simulink model "Sim5_MMC"  (R2019a)
settings: Solver=ode1  StartTime=0.0  StopTime=4  FixedStep=Time_Step  RelTol=1e-3
undefined symbols (not defined in the file): DiscIntNeverNeededParam, GRD00_Lg, GRD00_Rg, Time_Step, VSC01_id0
libraries: powerlib x107, Control_Lib x16, simulink x15, spsCurrentMeasurementLib x14, powerlib_meascontrol x4
(part 3 of 5)

== system Sim5_MMC/CCSC/Control loops/Power Control Loops ==
  P_mes : Inport
  P_set : Inport  Port=2
  delta_PLL : Inport  Port=3
  w_PLL : Inport  Port=4
  Compare To Constant : simulink/Logic and Bit Operations/Compare To Constant  relop===  const=1  OutDataTypeStr=boolean
  Compare To Constant1 : simulink/Logic and Bit Operations/Compare To Constant  relop===  const=2  OutDataTypeStr=boolean
  Compare To Constant2 : simulink/Logic and Bit Operations/Compare To Constant  relop===  const=3  OutDataTypeStr=boolean
  Inertia Less : Subsystem
  Multiport Switch : MultiPortSwitch
  Multiport Switch1 : MultiPortSwitch
  Mux : Mux  Inputs=[1 1]
  PI Controler : Subsystem
  Trigonometric Function : Trigonometry  Operator=cos
  Trigonometric Function1 : Trigonometry
  VSM : Subsystem
  w_set{1..4} (4 alike) : Constant  Value=Chosen_Strategy
  w_set_pu : Constant
  f : Outport  PortDimensions=1  VectorParamsAs1DForOutWhenUnconnected=off
  Theta : Outport  Port=2  VectorParamsAs1DForOutWhenUnconnected=off
  CosSinTheta : Outport  Port=3  PortDimensions=2  VectorParamsAs1DForOutWhenUnconnected=off
  wires:
  Multiport Switch1/1 -> Trigonometric Function1/1, Trigonometric Function/1, Theta/1
  Trigonometric Function1/1 -> Mux/2
  Mux/1 -> CosSinTheta/1
  Trigonometric Function/1 -> Mux/1
  Compare To Constant2/1 -> PI Controler/Enable
  Compare To Constant1/1 -> VSM/Enable
  Compare To Constant/1 -> Inertia Less/Enable
  w_set4/1 -> Compare To Constant2/1
  w_set2/1 -> Compare To Constant1/1
  w_set3/1 -> Compare To Constant/1
  Inertia Less/1(frequency) -> Multiport Switch/2
  Multiport Switch/1 -> f/1
  Inertia Less/2(theta) -> Multiport Switch1/2
  VSM/2(theta) -> Multiport Switch1/3
  w_set1/1 -> Multiport Switch/1, Multiport Switch1/1
  VSM/1(frequency) -> Multiport Switch/3
  PI Controler/1(frequency) -> Multiport Switch/4
  PI Controler/2(theta) -> Multiport Switch1/4
  w_set_pu/1 -> PI Controler/3(w_set_pu)
  w_PLL/1 -> Inertia Less/4(w_PLL), VSM/3(w_PLL)
  delta_PLL/1 -> Inertia Less/3(delta_PLL)
  P_set/1 -> Inertia Less/2(P_set), VSM/2(P_set), PI Controler/2(P_set)
  P_mes/1 -> Inertia Less/1(P_mes), VSM/1(P_mes), PI Controler/1(P_mes)

== system Sim5_MMC/CCSC/Control loops/Power Control Loops1 ==
  P_mes : Inport
  P_set : Inport  Port=2
  delta_PLL : Inport  Port=3
  w_PLL : Inport  Port=4
  Delta_E_dq : Inport  Port=5
  Compare To Constant : simulink/Logic and Bit Operations/Compare To Constant  relop===  const=1  OutDataTypeStr=boolean
  Compare To Constant1 : simulink/Logic and Bit Operations/Compare To Constant  relop===  const=2  OutDataTypeStr=boolean
  Compare To Constant2 : simulink/Logic and Bit Operations/Compare To Constant  relop===  const=3  OutDataTypeStr=boolean
  Inertia Less : Subsystem
  Multiport Switch : MultiPortSwitch
  Multiport Switch1 : MultiPortSwitch
  Mux : Mux  Inputs=[1 1]
  PI Controler : Subsystem
  Subsystem : Subsystem
  Trigonometric Function : Trigonometry  Operator=cos
  Trigonometric Function1 : Trigonometry
  VSM : Subsystem
  w_set{1..4} (4 alike) : Constant  Value=Chosen_Strategy
  w_set_pu : Constant
  f : Outport  PortDimensions=1  VectorParamsAs1DForOutWhenUnconnected=off
  Theta : Outport  Port=2  VectorParamsAs1DForOutWhenUnconnected=off
  CosSinTheta : Outport  Port=3  PortDimensions=2  VectorParamsAs1DForOutWhenUnconnected=off
  wires:
  Subsystem/1(Mod_h) -> PI Controler/3(Mod_H), VSM/3(Mod_H)
  Delta_E_dq/1 -> Subsystem/1(Delta_E_dq)
  Multiport Switch1/1 -> Trigonometric Function1/1, Trigonometric Function/1, Theta/1
  Trigonometric Function1/1 -> Mux/2
  Mux/1 -> CosSinTheta/1
  Trigonometric Function/1 -> Mux/1
  Compare To Constant2/1 -> PI Controler/Enable
  Compare To Constant1/1 -> VSM/Enable
  Compare To Constant/1 -> Inertia Less/Enable
  w_set4/1 -> Compare To Constant2/1
  w_set2/1 -> Compare To Constant1/1
  w_set3/1 -> Compare To Constant/1
  Inertia Less/1(frequency) -> Multiport Switch/2
  Multiport Switch/1 -> f/1
  Inertia Less/2(theta) -> Multiport Switch1/2
  VSM/2(theta) -> Multiport Switch1/3
  w_set1/1 -> Multiport Switch/1, Multiport Switch1/1
  VSM/1(frequency) -> Multiport Switch/3
  PI Controler/1(frequency) -> Multiport Switch/4
  PI Controler/2(theta) -> Multiport Switch1/4
  w_set_pu/1 -> PI Controler/4(w_set_pu)
  w_PLL/1 -> Inertia Less/4(w_PLL), VSM/4(w_PLL)
  delta_PLL/1 -> Inertia Less/3(delta_PLL)
  P_set/1 -> Inertia Less/2(P_set), VSM/2(P_set), PI Controler/2(P_set)
  P_mes/1 -> Inertia Less/1(P_mes), VSM/1(P_mes), PI Controler/1(P_mes)

== system Sim5_MMC/CCSC/Control loops/Subsystem ==
  Constant1 : Constant  Commented=on  Value=2*pi*50
  Constant2 : Constant  Commented=on  Value=[0 -2*pi/3 2*pi/3]
  Gain : Gain  Commented=on  Gain=sqrt(2)
  Gain1 : Gain  Commented=on  Gain=0.8
  Goto12 : Goto  Commented=on  GotoTag=Theta
  Integrator : Integrator  Commented=on
  Mux1 : Mux  Commented=on  Inputs=3
  Scope : Scope  Commented=on
  Sin : Trigonometry  Commented=on
  Sum2 : Sum  Commented=on  Inputs=|++
  wires:
  Gain1/1 -> Scope/1
  Mux1/1 -> Sum2/1
  Integrator/1 -> Mux1/3, Mux1/2, Mux1/1, Goto12/1
  Gain/1 -> Gain1/1
  Sin/1 -> Gain/1
  Sum2/1 -> Sin/1
  Constant2/1 -> Sum2/2
  Constant1/1 -> Integrator/1

== system Sim5_MMC/CCSC/Control loops/Transient Damping Resistance ==
  ig_dq : Inport
  Filter w_LF : Subsystem
      mask Display: disp('\omega_{LF} / (s + \omega_{LF})','texmode','on')
  Sum5 : Sum  Inputs=|+-
  nq1 : Gain  Gain=Rv
  "Delta_E_dq " : Outport  VectorParamsAs1DForOutWhenUnconnected=off
  wires:
  nq1/1 -> Filter w_LF/1(e), Sum5/2
  Filter w_LF/1(s) -> Sum5/1
  Sum5/1 -> "Delta_E_dq "/1
  ig_dq/1 -> nq1/1

== system Sim5_MMC/CCSC/Control loops/VI ==
  note: VI triggering and threshold computation
  note: VI
  i_VI_dq : Inport
  Demux1 : Demux  Outputs=2
      settings: DisplayOption=none
  Gain5 : Gain  Gain=DX_DR
  Gain6 : Gain  Gain=Kp_Rvi_pu
  Gain9 : Gain  Gain=DX_DR
  I_thresh : Constant
  Mux2 : Mux  Inputs=2
  Saturation : Saturate  UpperLimit=inf  LowerLimit=0
  Sum1 : Sum  Inputs=-+|
  Sum7 : Sum  Inputs=|+-
  Sum8 : Sum  Inputs=++|
  dq to phasor : Subsystem
  product{,1..3} (4 alike) : Product  InputSameDT=on  RndMeth=Zero  SaturateOnIntegerOverflow=on  OutDataTypeStr=Inherit: Same as first input
  I_rms : Outport  VectorParamsAs1DForOutWhenUnconnected=off
  Delta_E_dq : Outport  Port=2  VectorParamsAs1DForOutWhenUnconnected=off
  wires:
  Sum1/1 -> Saturation/1
  dq to phasor/1(rms) -> Sum1/2, I_rms/1  "I_rms"
  Saturation/1 -> Gain6/1
  I_thresh/1 -> Sum1/1
  Mux2/1 -> Delta_E_dq/1
  Gain6/1 -> product3/2, product/1, product1/2, product2/2
  product3/1 -> Gain5/1
  product/1 -> Gain9/1
  Demux1/1 -> product1/1, product/2  "igd"
  Demux1/2 -> product2/1, product3/1  "igq"
  product1/1 -> Sum7/1
  Gain5/1 -> Sum7/2
  Gain9/1 -> Sum8/1
  product2/1 -> Sum8/2
  Sum7/1 -> Mux2/1
  Sum8/1 -> Mux2/2
  i_VI_dq/1 -> dq to phasor/1(dq_mes), Demux1/1

== system Sim5_MMC/Energy Based/Bridge_Model/Decoupling voltage ==
  Vv_ref : Inport
  Vdiff_ref : Inport  Port=2
  Sum7 : Sum  Inputs=+-
  Sum8 : Sum
  Vmu_ref : Outport
  Vml_ref : Outport  Port=2
  wires:
  Sum8/1 -> Vml_ref/1  "Ul"
  Sum7/1 -> Vmu_ref/1
  Vdiff_ref/1 -> Sum8/1, Sum7/1
  Vv_ref/1 -> Sum8/2, Sum7/2

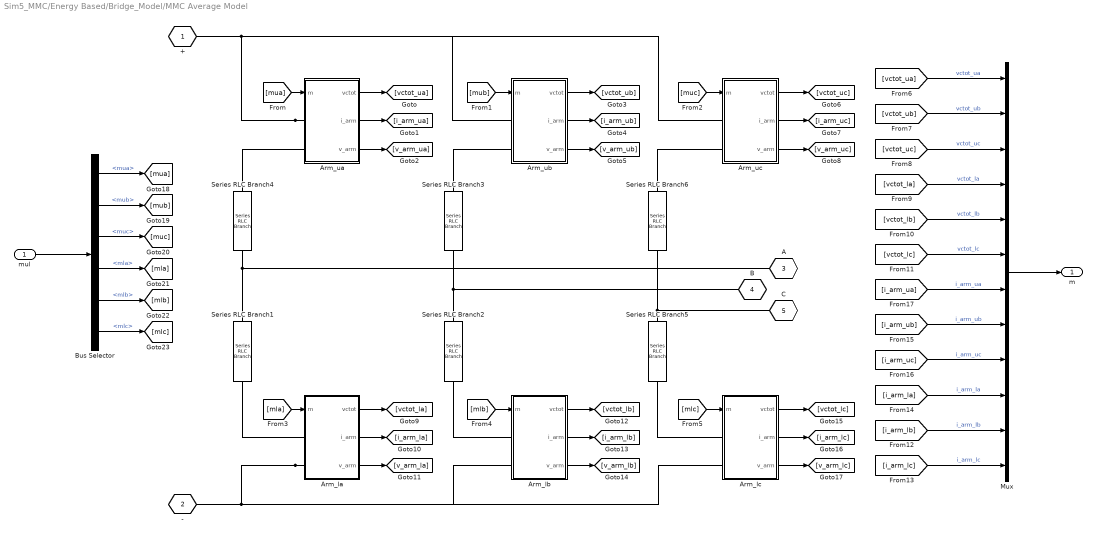
== system Sim5_MMC/Energy Based/Bridge_Model/MMC Average Model ==
  mul : Inport
  Arm_la : Subsystem  mask{C_arm=Carm, Vdc=Udcn}
      mask prompts: C_arm "Arm equivalent Capacitor (F)"; Vdc "Init DC Voltage (V)"
  Arm_lb : Subsystem  mask{C_arm=Carm, Vdc=Udcn}
      mask prompts: C_arm "Arm equivalent Capacitor (F)"; Vdc "Init DC Voltage (V)"
  Arm_lc : Subsystem  mask{C_arm=Carm, Vdc=Udcn}
      mask prompts: C_arm "Arm equivalent Capacitor (F)"; Vdc "Init DC Voltage (V)"
  Arm_ua : Subsystem  mask{C_arm=Carm, Vdc=Udcn}
      mask prompts: C_arm "Arm equivalent Capacitor (F)"; Vdc "Init DC Voltage (V)"
  Arm_ub : Subsystem  mask{C_arm=Carm, Vdc=Udcn}
      mask prompts: C_arm "Arm equivalent Capacitor (F)"; Vdc "Init DC Voltage (V)"
  Arm_uc : Subsystem  mask{C_arm=Carm, Vdc=Udcn}
      mask prompts: C_arm "Arm equivalent Capacitor (F)"; Vdc "Init DC Voltage (V)"
  Bus Selector : BusSelector  OutputSignals=mua,mub,muc,mla,mlb,mlc
  Mux : Mux  Inputs=12
  Series RLC Branch{1..6} (6 alike) : powerlib/Elements/Series RLC Branch  LConnTagsString=__new0  RConnTagsString=__new0  BranchType=RL  Resistance=Rarm_pu*Zb  Inductance=Larm_pu*Lb  SetiL0=off  InitialCurrent=0  Capacitance=1e-6  Setx0=off  InitialVoltage=0  Measurements=None
  + : PMIOPort  Tag=PMCPort  Side=Right
  - : PMIOPort  Tag=PMCPort  Port=2  Side=Right
  A : PMIOPort  Tag=PMCPort  Port=3  Side=Left
  B : PMIOPort  Tag=PMCPort  Port=4  Side=Left
  C : PMIOPort  Tag=PMCPort  Port=5  Side=Left
  m : Outport
  wires:
  [mlb] -> Arm_lb/1(m)
  [mlc] -> Arm_lc/1(m)
  [mla] -> Arm_la/1(m)
  Arm_uc/1(vctot) -> [vctot_uc]
  Arm_lb/3(v_arm) -> [v_arm_lb]
  Arm_ub/3(v_arm) -> [v_arm_ub]
  Arm_ua/1(vctot) -> [vctot_ua]
  Arm_uc/2(i_arm) -> [i_arm_uc]
  Arm_lc/1(vctot) -> [vctot_lc]
  Arm_la/2(i_arm) -> [i_arm_la]
  Arm_la/1(vctot) -> [vctot_la]
  Arm_ub/2(i_arm) -> [i_arm_ub]
  Arm_lc/3(v_arm) -> [v_arm_lc]
  Arm_la/3(v_arm) -> [v_arm_la]
  [mua] -> Arm_ua/1(m)
  Arm_ub/1(vctot) -> [vctot_ub]
  Arm_lb/1(vctot) -> [vctot_lb]
  [mub] -> Arm_ub/1(m)
  Arm_uc/3(v_arm) -> [v_arm_uc]
  Arm_lb/2(i_arm) -> [i_arm_lb]
  Arm_ua/2(i_arm) -> [i_arm_ua]
  Arm_lc/2(i_arm) -> [i_arm_lc]
  [muc] -> Arm_uc/1(m)
  Arm_ua/3(v_arm) -> [v_arm_ua]
  mul/1 -> Bus Selector/1
  Bus Selector/1 -> [mua]  "<mua>"
  Bus Selector/2 -> [mub]  "<mub>"
  Bus Selector/3 -> [muc]  "<muc>"
  Bus Selector/6 -> [mlc]  "<mlc>"
  Bus Selector/5 -> [mlb]  "<mlb>"
  Bus Selector/4 -> [mla]  "<mla>"
  [vctot_lc] -> Mux/6  "vctot_lc"
  [vctot_uc] -> Mux/3  "vctot_uc"
  [i_arm_ua] -> Mux/7  "i_arm_ua"
  [i_arm_ub] -> Mux/8  "i_arm_ub"
  [vctot_lb] -> Mux/5  "vctot_lb"
  [i_arm_la] -> Mux/10  "i_arm_la"
  [vctot_ub] -> Mux/2  "vctot_ub"
  [i_arm_uc] -> Mux/9  "i_arm_uc"
  [vctot_la] -> Mux/4  "vctot_la"
  [i_arm_lb] -> Mux/11  "i_arm_lb"
  [vctot_ua] -> Mux/1  "vctot_ua"
  [i_arm_lc] -> Mux/12  "i_arm_lc"
  Mux/1 -> m/1
  connections:
  Series RLC Branch5/RConn1 -- Arm_lc/LConn1
  Arm_ua/LConn2 -- Series RLC Branch4/LConn1
  Series RLC Branch6/LConn1 -- Arm_uc/LConn2
  Series RLC Branch5/LConn1 -- Series RLC Branch6/RConn1 -- C/RConn1
  Series RLC Branch2/LConn1 -- B/RConn1 -- Series RLC Branch3/RConn1
  Arm_ub/LConn2 -- Series RLC Branch3/LConn1
  Series RLC Branch2/RConn1 -- Arm_lb/LConn1
  Series RLC Branch1/LConn1 -- Series RLC Branch4/RConn1 -- A/RConn1
  Arm_la/LConn2 -- -/RConn1 -- Arm_lc/LConn2 -- Arm_lb/LConn2
  Series RLC Branch1/RConn1 -- Arm_la/LConn1
  Arm_ua/LConn1 -- +/RConn1 -- Arm_uc/LConn1 -- Arm_ub/LConn1

== system Sim5_MMC/Energy Based/Bridge_Model/Modulation Index Generation ==
  vmu_ref : Inport
  vml_ref : Inport  Port=2
  "1 -> Activer filtre notch 0 -> Désactiver filtre notch2" : Constant  Value=Udcn
  Bus Creator : BusCreator  Inputs=6
  Demux : Demux  Outputs=3
  Demux1 : Demux  Outputs=3
  Demux2 : Demux  Outputs=[3 3]
  Divide1 : Product  Inputs=/*
  Divide4 : Product  Inputs=*/
  Manual Switch : ManualSwitch
  Manual Switch1 : ManualSwitch  CurrentSetting=0
  Selector : Selector  InputPortWidth=12  IndexOptions=Index vector (dialog)  Indices=[1 2 3 4 5 6]  OutputSizes=1
  m limiter low : Saturate  UpperLimit=1  LowerLimit=0
  m limiter up : Saturate  UpperLimit=1  LowerLimit=0
  mul : Outport
  wires:
  Demux/3 -> Bus Creator/3  "muc"
  vmu_ref/1 -> Divide1/2
  Manual Switch/1 -> Divide1/1
  Bus Creator/1 -> mul/1
  Demux1/1 -> Bus Creator/4  "mla"
  Demux1/2 -> Bus Creator/5  "mlb"
  Divide4/1 -> m limiter low/1
  Demux1/3 -> Bus Creator/6  "mlc"
  Manual Switch1/1 -> Divide4/2
  Demux/2 -> Bus Creator/2  "mub"
  vml_ref/1 -> Divide4/1
  Demux/1 -> Bus Creator/1  "mua"
  m limiter up/1 -> Demux/1
  Divide1/1 -> m limiter up/1
  m limiter low/1 -> Demux1/1
  "1 -> Activer filtre notch 0 -> Désactiver filtre notch2"/1 -> Manual Switch/2, Manual Switch1/1
  Selector/1 -> Demux2/1
  [m_mmc] -> Selector/1
  Demux2/1 -> Manual Switch/1
  Demux2/2 -> Manual Switch1/2

== system Sim5_MMC/Energy Based/Control loops/ pu P//Q computation ==
  v_abc_pu : Inport  PortDimensions=3
  i_abc_pu : Inport  Port=2  PortDimensions=3
  Demux : Demux  Outputs=3
      settings: DisplayOption=none
  Mux : Mux  Inputs=3
  Product1 : Product  InputSameDT=on  SaturateOnIntegerOverflow=on  OutDataTypeStr=Inherit: Same as first input
  Product3 : Product  InputSameDT=on  SaturateOnIntegerOverflow=on  OutDataTypeStr=Inherit: Same as first input
  Sum : Sum  Inputs=+-  InputSameDT=on  SaturateOnIntegerOverflow=on  OutDataTypeStr=Inherit: Same as first input
  Sum1 : Sum  Inputs=1  InputSameDT=on  SaturateOnIntegerOverflow=on  OutDataTypeStr=Inherit: Same as first input
  Sum4 : Sum  Inputs=1  InputSameDT=on  SaturateOnIntegerOverflow=on  OutDataTypeStr=Inherit: Same as first input
  Sum5 : Sum  Inputs=+-  InputSameDT=on  SaturateOnIntegerOverflow=on  OutDataTypeStr=Inherit: Same as first input
  Sum6 : Sum  Inputs=+-  InputSameDT=on  SaturateOnIntegerOverflow=on  OutDataTypeStr=Inherit: Same as first input
  pu->V : Gain  Gain=1/sqrt(3)  SaturateOnIntegerOverflow=on  OutDataTypeStr=Inherit: Same as input  ParamDataTypeStr=Inherit: Same as input
  pu->V1 : Gain  Gain=1/3  SaturateOnIntegerOverflow=on  OutDataTypeStr=Inherit: Same as input  ParamDataTypeStr=Inherit: Same as input
  pu->V2 : Gain  Gain=1/3  SaturateOnIntegerOverflow=on  OutDataTypeStr=Inherit: Same as input  ParamDataTypeStr=Inherit: Same as input
  P : Outport  VectorParamsAs1DForOutWhenUnconnected=off
  Q : Outport  Port=2  VectorParamsAs1DForOutWhenUnconnected=off
  wires:
  pu->V2/1 -> Q/1
  pu->V1/1 -> P/1
  Sum1/1 -> pu->V/1
  Product3/1 -> Sum1/1
  Product1/1 -> Sum4/1
  v_abc_pu/1 -> Product1/1, Demux/1
  i_abc_pu/1 -> Product1/2, Product3/2
  Sum4/1 -> pu->V1/1
  Demux/1 -> Sum/1, Sum6/2
  Demux/2 -> Sum/2, Sum5/1
  Demux/3 -> Sum5/2, Sum6/1
  Sum/1 -> Mux/3
  Sum5/1 -> Mux/1
  Sum6/1 -> Mux/2
  Mux/1 -> Product3/1
  pu->V/1 -> pu->V2/1  "Q"

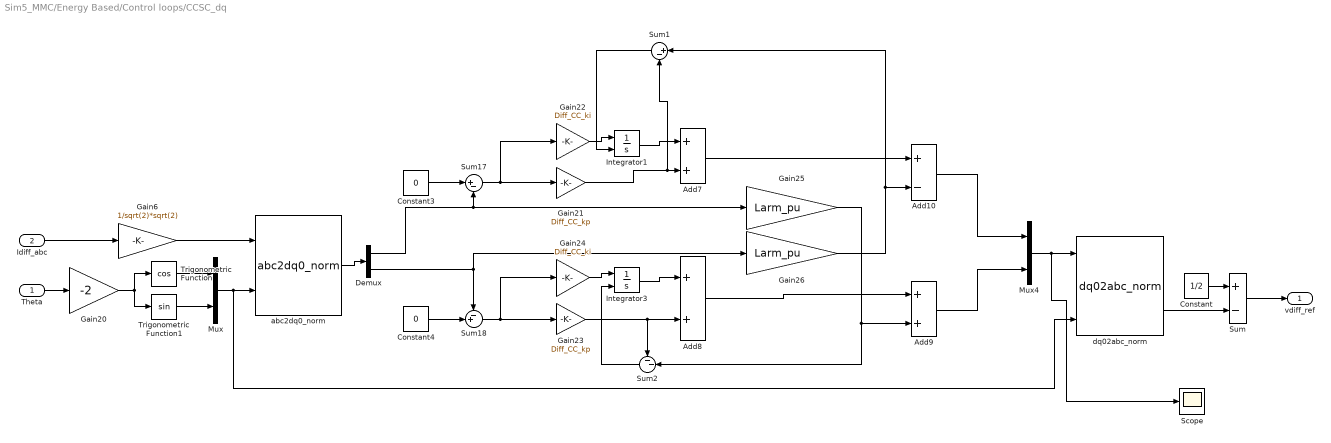
== system Sim5_MMC/Energy Based/Control loops/CCSC_dq ==
  Theta : Inport
  Idiff_abc : Inport  Port=2
  Add10 : Sum  Inputs=+-
  Add7 : Sum
  Add8 : Sum
  Add9 : Sum
  Constant : Constant  Value=1/2
  Constant3 : Constant  Value=0
  Constant4 : Constant  Value=0
  Demux : Demux  Outputs=2
  Gain20 : Gain  Gain=-2
  Gain21 : Gain  Gain=Diff_CC_kp
  Gain22 : Gain  Gain=Diff_CC_ki
  Gain23 : Gain  Gain=Diff_CC_kp
  Gain24 : Gain  Gain=Diff_CC_ki
  Gain25 : Gain  Gain=Larm_pu
  Gain26 : Gain  Gain=Larm_pu
  Gain6 : Gain  Gain=1/sqrt(2)*sqrt(2)
  Integrator1 : Integrator  InitialConditionSource=external
  Integrator3 : Integrator  InitialConditionSource=external
  Mux : Mux  Inputs=2
  Mux4 : Mux  Inputs=2
  Scope : Scope
  Sum : Sum  Inputs=+-
  Sum1 : Sum  Inputs=|+-
  Sum17 : Sum  Inputs=|+-
  Sum18 : Sum  Inputs=-+|
  Sum2 : Sum  Inputs=--|
  Trigonometric Function : Trigonometry  Operator=cos
  Trigonometric Function1 : Trigonometry
  abc2dq0_norm : Control_Lib/abc2dq0_norm  referenceAxisMode=Reference axis at 90 degrees behind phase_a  baseUpdateGain=1/sqrt(3)
      settings: SourceProductName=VSC4SPS
  dq02abc_norm : Control_Lib/dq02abc_norm  referenceAxisMode=Reference axis at 90 degrees behind phase_a  baseUpdateGain=sqrt(3)
      settings: SourceProductName=VSC4SPS
  vdiff_ref : Outport
  wires:
  Theta/1 -> Gain20/1
  Constant3/1 -> Sum17/1
  Demux/2 -> Sum18/1, Gain26/1
  Add7/1 -> Add10/1
  Gain24/1 -> Integrator3/1
  Add8/1 -> Add9/1
  Idiff_abc/1 -> Gain6/1
  Sum17/1 -> Gain22/1, Gain21/1
  Gain21/1 -> Sum1/2, Add7/2
  Gain23/1 -> Sum2/1, Add8/2
  Add9/1 -> Mux4/2
  Sum18/1 -> Gain23/1, Gain24/1
  Constant4/1 -> Sum18/2
  Add10/1 -> Mux4/1
  Integrator3/1 -> Add8/1
  Mux/1 -> dq02abc_norm/3, abc2dq0_norm/2
  Gain22/1 -> Integrator1/1
  Gain25/1 -> Sum2/2, Add9/2
  Demux/1 -> Gain25/1, Sum17/2
  Integrator1/1 -> Add7/1
  Gain26/1 -> Sum1/1, Add10/2
  dq02abc_norm/2 -> Sum/2
  Gain6/1 -> abc2dq0_norm/1
  Trigonometric Function/1 -> Mux/1
  Gain20/1 -> Trigonometric Function1/1, Trigonometric Function/1
  Trigonometric Function1/1 -> Mux/2
  abc2dq0_norm/2 -> Demux/1
  Mux4/1 -> Scope/1, dq02abc_norm/1
  Sum/1 -> vdiff_ref/1
  Constant/1 -> Sum/1
  Sum1/1 -> Integrator1/2
  Sum2/1 -> Integrator3/2

== system Sim5_MMC/Energy Based/Control loops/Current Limitation ==
  note: Current limitation
  Vm_dq* : Inport
  Ig_dq : Inport  Port=2
  vg_dq : Inport  Port=3
  Constant : Constant  Value=I_max_pu
  Current control : Subsystem
  Demux : Demux  Outputs=2
  Demux2 : Demux  Outputs=2
  Inverse Current control : Subsystem
  Mux : Mux  Inputs=2
  Product{,1..3} (4 alike) : Product
  Saturation Dynamic : simulink/Discontinuities/Saturation Dynamic  OutMin=[]  OutMax=[]  OutDataTypeStr=Inherit: Same as second input  OutDataType=fixdt(1, 16)  OutScaling=2^-10  DoSatur=off
  Sqrt : Sqrt  SaturateOnIntegerOverflow=on
  Sum : Sum
  Trigonometric Function : Trigonometry  Operator=atan2  NumberOfIterations=5  OutputSignalType=real
  Trigonometric Function1 : Trigonometry  Operator=cos
  Trigonometric Function2 : Trigonometry
  w_set1 : Constant
  w_set2 : Constant
  w_set3 : Constant  Value=0
  Vm_dq_sat : Outport  VectorParamsAs1DForOutWhenUnconnected=off
  wires:
  w_set3/1 -> Saturation Dynamic/3
  Constant/1 -> Saturation Dynamic/1
  Mux/1 -> Current control/1(Ig_dq0*)
  Product/1 -> Mux/1
  Demux/1 -> Product1/1, Product1/2
  Demux/2 -> Product2/1, Product2/2
  Trigonometric Function2/1 -> Product3/2
  Product2/1 -> Sum/2
  Trigonometric Function1/1 -> Product/2
  Demux2/1 -> Trigonometric Function/2
  Trigonometric Function/1 -> Trigonometric Function2/1, Trigonometric Function1/1
  Saturation Dynamic/1 -> Product/1, Product3/1
  Product1/1 -> Sum/1
  Sqrt/1 -> Saturation Dynamic/2
  Demux2/2 -> Trigonometric Function/1
  Inverse Current control/1(Is_dq*) -> Demux2/1, Demux/1
  Sum/1 -> Sqrt/1
  Product3/1 -> Mux/2
  Ig_dq/1 -> Inverse Current control/2(Ig_dq), Current control/2(Ig_dq0)
  w_set1/1 -> Inverse Current control/4(w)
  w_set2/1 -> Current control/4(w)
  vg_dq/1 -> Current control/3(vg_dq0), Inverse Current control/3(vg_dq)
  Vm_dq*/1 -> Inverse Current control/1(Vm_dq*)
  Current control/1(vm) -> Vm_dq_sat/1

== system Sim5_MMC/Energy Based/Control loops/DC part: stored energy control + differential current control ==
  Wtot_ref_pu : Inport
  theta : Inport  Port=2
  vctot_up_pu : Inport  Port=3
  vctot_low_pu : Inport  Port=4
  Vdc_pu : Inport  Port=5
  pac_pu : Inport  Port=6
  idff_pu : Inport  Port=7
  vv_pu : Inport  Port=8
  Constant : Constant  Value=[0 0 0]  SampleTime=-1
  Control Wdiff : Subsystem
  "Control Wtot " : Subsystem
  Differential_current_control : Subsystem
  Sum5 : Sum
  Wdiff computation : Subsystem
  Wtot computation : Subsystem
  vdiff_pu_ref : Outport  PortDimensions=3
  wires:
  Vdc_pu/1 -> "Control Wtot "/4(Vdc_pu), Differential_current_control/1(vdc_pu)
  Wtot_ref_pu/1 -> "Control Wtot "/2(Wtot ref pu)
  "Control Wtot "/1(Idiff ref pu) -> Sum5/1
  idff_pu/1 -> Differential_current_control/2(idiff_pu)
  Sum5/1 -> Differential_current_control/3(idiff_ref_pu)
  vctot_up_pu/1 -> Wdiff computation/1(vctot u_pu), Wtot computation/1(vctot u_pu)
  vctot_low_pu/1 -> Wdiff computation/2(vctot l_pu), Wtot computation/2(vctot l_pu)
  Wdiff computation/1(Wdiff) -> Control Wdiff/1(Wdiff pu)
  Wtot computation/1(Wtot) -> "Control Wtot "/1(Wtot_pu)
  theta/1 -> Control Wdiff/3(theta)
  Constant/1 -> Control Wdiff/2(Wdiff_ref pu)
  Differential_current_control/1(Vprediff_ref_pu) -> vdiff_pu_ref/1
  pac_pu/1 -> "Control Wtot "/3(p_ac_pu)
  Control Wdiff/2(Idiff ref pu1) -> Sum5/2
  vv_pu/1 -> Control Wdiff/4(vv_pu)

== system Sim5_MMC/Energy Based/Control loops/Power Control Loops1 ==
  P_mes : Inport
  P_set : Inport  Port=2
  delta_PLL : Inport  Port=3
  w_PLL : Inport  Port=4
  Delta_E_dq : Inport  Port=5
  Compare To Constant : simulink/Logic and Bit Operations/Compare To Constant  relop===  const=1  OutDataTypeStr=boolean
  Compare To Constant1 : simulink/Logic and Bit Operations/Compare To Constant  relop===  const=2  OutDataTypeStr=boolean
  Compare To Constant2 : simulink/Logic and Bit Operations/Compare To Constant  relop===  const=3  OutDataTypeStr=boolean
  Inertia Less : Subsystem
  Multiport Switch : MultiPortSwitch
  Multiport Switch1 : MultiPortSwitch
  Mux : Mux  Inputs=[1 1]
  PI Controler : Subsystem
  Subsystem : Subsystem
  Trigonometric Function : Trigonometry  Operator=cos
  Trigonometric Function1 : Trigonometry
  VSM : Subsystem
  w_set{1..4} (4 alike) : Constant  Value=Chosen_Strategy
  w_set_pu : Constant
  f : Outport  PortDimensions=1  VectorParamsAs1DForOutWhenUnconnected=off
  Theta : Outport  Port=2  VectorParamsAs1DForOutWhenUnconnected=off
  CosSinTheta : Outport  Port=3  PortDimensions=2  VectorParamsAs1DForOutWhenUnconnected=off
  wires:
  Subsystem/1(Mod_h) -> PI Controler/3(Mod_H), VSM/3(Mod_H)
  Delta_E_dq/1 -> Subsystem/1(Delta_E_dq)
  Multiport Switch1/1 -> Trigonometric Function1/1, Trigonometric Function/1, Theta/1
  Trigonometric Function1/1 -> Mux/2
  Mux/1 -> CosSinTheta/1
  Trigonometric Function/1 -> Mux/1
  Compare To Constant2/1 -> PI Controler/Enable
  Compare To Constant1/1 -> VSM/Enable
  Compare To Constant/1 -> Inertia Less/Enable
  w_set4/1 -> Compare To Constant2/1
  w_set2/1 -> Compare To Constant1/1
  w_set3/1 -> Compare To Constant/1
  Inertia Less/1(frequency) -> Multiport Switch/2
  Multiport Switch/1 -> f/1
  Inertia Less/2(theta) -> Multiport Switch1/2
  VSM/2(theta) -> Multiport Switch1/3
  w_set1/1 -> Multiport Switch/1, Multiport Switch1/1
  VSM/1(frequency) -> Multiport Switch/3
  PI Controler/1(frequency) -> Multiport Switch/4
  PI Controler/2(theta) -> Multiport Switch1/4
  w_set_pu/1 -> PI Controler/4(w_set_pu)
  w_PLL/1 -> Inertia Less/4(w_PLL), VSM/4(w_PLL)
  delta_PLL/1 -> Inertia Less/3(delta_PLL)
  P_set/1 -> Inertia Less/2(P_set), VSM/2(P_set), PI Controler/2(P_set)
  P_mes/1 -> Inertia Less/1(P_mes), VSM/1(P_mes), PI Controler/1(P_mes)

== system Sim5_MMC/Energy Based/Control loops/Subsystem ==
  Constant1 : Constant  Commented=on  Value=2*pi*50
  Constant2 : Constant  Commented=on  Value=[0 -2*pi/3 2*pi/3]
  Gain : Gain  Commented=on  Gain=sqrt(2)
  Gain1 : Gain  Commented=on  Gain=0.8
  Goto12 : Goto  Commented=on  GotoTag=Theta
  Integrator : Integrator  Commented=on
  Mux1 : Mux  Commented=on  Inputs=3
  Scope : Scope  Commented=on
  Sin : Trigonometry  Commented=on
  Sum2 : Sum  Commented=on  Inputs=|++
  wires:
  Gain1/1 -> Scope/1
  Mux1/1 -> Sum2/1
  Integrator/1 -> Mux1/3, Mux1/2, Mux1/1, Goto12/1
  Gain/1 -> Gain1/1
  Sin/1 -> Gain/1
  Sum2/1 -> Sin/1
  Constant2/1 -> Sum2/2
  Constant1/1 -> Integrator/1

== system Sim5_MMC/Energy Based/Control loops/Transient Damping Resistance ==
  ig_dq : Inport
  Filter w_LF : Subsystem
      mask Display: disp('\omega_{LF} / (s + \omega_{LF})','texmode','on')
  Sum5 : Sum  Inputs=|+-
  nq1 : Gain  Gain=Rv
  "Delta_E_dq " : Outport  VectorParamsAs1DForOutWhenUnconnected=off
  wires:
  nq1/1 -> Filter w_LF/1(e), Sum5/2
  Filter w_LF/1(s) -> Sum5/1
  Sum5/1 -> "Delta_E_dq "/1
  ig_dq/1 -> nq1/1

== system Sim5_MMC/Energy Based/Control loops/VI ==
  note: VI triggering and threshold computation
  note: VI
  i_VI_dq : Inport
  Demux1 : Demux  Outputs=2
      settings: DisplayOption=none
  Gain5 : Gain  Gain=DX_DR
  Gain6 : Gain  Gain=Kp_Rvi_pu
  Gain9 : Gain  Gain=DX_DR
  I_thresh : Constant  Value=I_thresh_pu
  Mux2 : Mux  Inputs=2
  Saturation : Saturate  UpperLimit=inf  LowerLimit=0
  Sum1 : Sum  Inputs=-+|
  Sum7 : Sum  Inputs=|+-
  Sum8 : Sum  Inputs=++|
  dq to phasor : Subsystem
  product{,1..3} (4 alike) : Product  InputSameDT=on  RndMeth=Zero  SaturateOnIntegerOverflow=on  OutDataTypeStr=Inherit: Same as first input
  I_rms : Outport  VectorParamsAs1DForOutWhenUnconnected=off
  Delta_E_dq : Outport  Port=2  VectorParamsAs1DForOutWhenUnconnected=off
  wires:
  Sum1/1 -> Saturation/1
  dq to phasor/1(rms) -> Sum1/2, I_rms/1  "I_rms"
  Saturation/1 -> Gain6/1
  I_thresh/1 -> Sum1/1
  Mux2/1 -> Delta_E_dq/1
  Gain6/1 -> product3/2, product/1, product1/2, product2/2
  product3/1 -> Gain5/1
  product/1 -> Gain9/1
  Demux1/1 -> product1/1, product/2  "igd"
  Demux1/2 -> product2/1, product3/1  "igq"
  product1/1 -> Sum7/1
  Gain5/1 -> Sum7/2
  Gain9/1 -> Sum8/1
  product2/1 -> Sum8/2
  Sum7/1 -> Mux2/1
  Sum8/1 -> Mux2/2
  i_VI_dq/1 -> dq to phasor/1(dq_mes), Demux1/1

== system Sim5_MMC/Mean Model 2-Level L-filter/Control loops/ pu P//Q computation ==
  v_abc_pu : Inport  PortDimensions=3
  i_abc_pu : Inport  Port=2  PortDimensions=3
  Demux : Demux  Outputs=3
      settings: DisplayOption=none
  Mux : Mux  Inputs=3
  Product1 : Product  InputSameDT=on  SaturateOnIntegerOverflow=on  OutDataTypeStr=Inherit: Same as first input
  Product3 : Product  InputSameDT=on  SaturateOnIntegerOverflow=on  OutDataTypeStr=Inherit: Same as first input
  Sum : Sum  Inputs=+-  InputSameDT=on  SaturateOnIntegerOverflow=on  OutDataTypeStr=Inherit: Same as first input
  Sum1 : Sum  Inputs=1  InputSameDT=on  SaturateOnIntegerOverflow=on  OutDataTypeStr=Inherit: Same as first input
  Sum4 : Sum  Inputs=1  InputSameDT=on  SaturateOnIntegerOverflow=on  OutDataTypeStr=Inherit: Same as first input
  Sum5 : Sum  Inputs=+-  InputSameDT=on  SaturateOnIntegerOverflow=on  OutDataTypeStr=Inherit: Same as first input
  Sum6 : Sum  Inputs=+-  InputSameDT=on  SaturateOnIntegerOverflow=on  OutDataTypeStr=Inherit: Same as first input
  pu->V : Gain  Gain=1/sqrt(3)  SaturateOnIntegerOverflow=on  OutDataTypeStr=Inherit: Same as input  ParamDataTypeStr=Inherit: Same as input
  pu->V1 : Gain  Gain=1/3  SaturateOnIntegerOverflow=on  OutDataTypeStr=Inherit: Same as input  ParamDataTypeStr=Inherit: Same as input
  pu->V2 : Gain  Gain=1/3  SaturateOnIntegerOverflow=on  OutDataTypeStr=Inherit: Same as input  ParamDataTypeStr=Inherit: Same as input
  P : Outport  VectorParamsAs1DForOutWhenUnconnected=off
  Q : Outport  Port=2  VectorParamsAs1DForOutWhenUnconnected=off
  wires:
  pu->V2/1 -> Q/1
  pu->V1/1 -> P/1
  Sum1/1 -> pu->V/1
  Product3/1 -> Sum1/1
  Product1/1 -> Sum4/1
  v_abc_pu/1 -> Product1/1, Demux/1
  i_abc_pu/1 -> Product1/2, Product3/2
  Sum4/1 -> pu->V1/1
  Demux/1 -> Sum/1, Sum6/2
  Demux/2 -> Sum/2, Sum5/1
  Demux/3 -> Sum5/2, Sum6/1
  Sum/1 -> Mux/3
  Sum5/1 -> Mux/1
  Sum6/1 -> Mux/2
  Mux/1 -> Product3/1
  pu->V/1 -> pu->V2/1  "Q"

== system Sim5_MMC/Mean Model 2-Level L-filter/Control loops/Current Limitation ==
  note: Current limitation
  Vm_dq* : Inport
  Ig_dq : Inport  Port=2
  vg_dq : Inport  Port=3
  Constant : Constant  Value=I_max_pu
  Current control : Subsystem
  Demux : Demux  Outputs=2
  Demux2 : Demux  Outputs=2
  Inverse Current control : Subsystem
  Mux : Mux  Inputs=2
  Product{,1..3} (4 alike) : Product
  Saturation Dynamic : simulink/Discontinuities/Saturation Dynamic  OutMin=[]  OutMax=[]  OutDataTypeStr=Inherit: Same as second input  OutDataType=fixdt(1, 16)  OutScaling=2^-10  DoSatur=off
  Sqrt : Sqrt  SaturateOnIntegerOverflow=on
  Sum : Sum
  Trigonometric Function : Trigonometry  Operator=atan2  NumberOfIterations=5  OutputSignalType=real
  Trigonometric Function1 : Trigonometry  Operator=cos
  Trigonometric Function2 : Trigonometry
  w_set1 : Constant
  w_set2 : Constant
  w_set3 : Constant  Value=0
  Vm_dq_sat : Outport  VectorParamsAs1DForOutWhenUnconnected=off
  wires:
  w_set3/1 -> Saturation Dynamic/3
  Constant/1 -> Saturation Dynamic/1
  Mux/1 -> Current control/1(Ig_dq0*)
  Product/1 -> Mux/1
  Demux/1 -> Product1/1, Product1/2
  Demux/2 -> Product2/1, Product2/2
  Trigonometric Function2/1 -> Product3/2
  Product2/1 -> Sum/2
  Trigonometric Function1/1 -> Product/2
  Demux2/1 -> Trigonometric Function/2
  Trigonometric Function/1 -> Trigonometric Function2/1, Trigonometric Function1/1
  Saturation Dynamic/1 -> Product/1, Product3/1
  Product1/1 -> Sum/1
  Sqrt/1 -> Saturation Dynamic/2
  Demux2/2 -> Trigonometric Function/1
  Inverse Current control/1(Is_dq*) -> Demux2/1, Demux/1
  Sum/1 -> Sqrt/1
  Product3/1 -> Mux/2
  Ig_dq/1 -> Inverse Current control/2(Ig_dq), Current control/2(Ig_dq0)
  w_set1/1 -> Inverse Current control/4(w)
  w_set2/1 -> Current control/4(w)
  vg_dq/1 -> Current control/3(vg_dq0), Inverse Current control/3(vg_dq)
  Vm_dq*/1 -> Inverse Current control/1(Vm_dq*)
  Current control/1(vm) -> Vm_dq_sat/1

== system Sim5_MMC/Mean Model 2-Level L-filter/Control loops/Power Control Loops ==
  P_mes : Inport
  P_set : Inport  Port=2
  delta_PLL : Inport  Port=3
  w_PLL : Inport  Port=4
  Delta_E_dq : Inport  Port=5
  Compare To Constant : simulink/Logic and Bit Operations/Compare To Constant  relop===  const=1  OutDataTypeStr=boolean
  Compare To Constant1 : simulink/Logic and Bit Operations/Compare To Constant  relop===  const=2  OutDataTypeStr=boolean
  Compare To Constant2 : simulink/Logic and Bit Operations/Compare To Constant  relop===  const=3  OutDataTypeStr=boolean
  Inertia Less : Subsystem
  Multiport Switch : MultiPortSwitch
  Multiport Switch1 : MultiPortSwitch
  Mux : Mux  Inputs=[1 1]
  PI Controler : Subsystem
  Subsystem : Subsystem
  Trigonometric Function : Trigonometry  Operator=cos
  Trigonometric Function1 : Trigonometry
  VSM : Subsystem
  w_set{1..4} (4 alike) : Constant  Value=Chosen_Strategy
  w_set_pu : Constant
  f : Outport  PortDimensions=1  VectorParamsAs1DForOutWhenUnconnected=off
  Theta : Outport  Port=2  VectorParamsAs1DForOutWhenUnconnected=off
  CosSinTheta : Outport  Port=3  PortDimensions=2  VectorParamsAs1DForOutWhenUnconnected=off
  wires:
  Subsystem/1(Mod_h) -> PI Controler/3(Mod_H), VSM/3(Mod_H)
  Delta_E_dq/1 -> Subsystem/1(Delta_E_dq)
  Multiport Switch1/1 -> Trigonometric Function1/1, Trigonometric Function/1, Theta/1
  Trigonometric Function1/1 -> Mux/2
  Mux/1 -> CosSinTheta/1
  Trigonometric Function/1 -> Mux/1
  Compare To Constant2/1 -> PI Controler/Enable
  Compare To Constant1/1 -> VSM/Enable
  Compare To Constant/1 -> Inertia Less/Enable
  w_set4/1 -> Compare To Constant2/1
  w_set2/1 -> Compare To Constant1/1
  w_set3/1 -> Compare To Constant/1
  Inertia Less/1(frequency) -> Multiport Switch/2
  Multiport Switch/1 -> f/1
  Inertia Less/2(theta) -> Multiport Switch1/2
  VSM/2(theta) -> Multiport Switch1/3
  w_set1/1 -> Multiport Switch/1, Multiport Switch1/1
  VSM/1(frequency) -> Multiport Switch/3
  PI Controler/1(frequency) -> Multiport Switch/4
  PI Controler/2(theta) -> Multiport Switch1/4
  w_set_pu/1 -> PI Controler/4(w_set_pu)
  w_PLL/1 -> Inertia Less/4(w_PLL), VSM/4(w_PLL)
  delta_PLL/1 -> Inertia Less/3(delta_PLL)
  P_set/1 -> Inertia Less/2(P_set), VSM/2(P_set), PI Controler/2(P_set)
  P_mes/1 -> Inertia Less/1(P_mes), VSM/1(P_mes), PI Controler/1(P_mes)

== system Sim5_MMC/Mean Model 2-Level L-filter/Control loops/RMS derivation ==
  dq : Inport
  Demux : Demux  Outputs=2
  Sqrt : Sqrt  SaturateOnIntegerOverflow=on
  Square : Math  Operator=square  SaturateOnIntegerOverflow=on
  Square1 : Math  Operator=square  SaturateOnIntegerOverflow=on
  Sum : Sum
  rms : Outport
  wires:
  dq/1 -> Demux/1
  Demux/2 -> Square1/1
  Square/1 -> Sum/1
  Demux/1 -> Square/1
  Sqrt/1 -> rms/1
  Sum/1 -> Sqrt/1
  Square1/1 -> Sum/2

== system Sim5_MMC/Mean Model 2-Level L-filter/Control loops/Transient Damping Resistance ==
  ig_dq : Inport
  Filter w_LF : Subsystem
      mask Display: disp('\omega_{LF} / (s + \omega_{LF})','texmode','on')
  Sum5 : Sum  Inputs=|+-
  nq1 : Gain  Gain=Rv
  "Delta_E_dq " : Outport  VectorParamsAs1DForOutWhenUnconnected=off
  wires:
  nq1/1 -> Filter w_LF/1(e), Sum5/2
  Filter w_LF/1(s) -> Sum5/1
  Sum5/1 -> "Delta_E_dq "/1
  ig_dq/1 -> nq1/1

== system Sim5_MMC/Mean Model 2-Level L-filter/Control loops/VI ==
  note: VI triggering and threshold computation
  note: VI
  i_VI_dq : Inport
  Demux1 : Demux  Outputs=2
      settings: DisplayOption=none
  Gain5 : Gain  Gain=DX_DR
  Gain6 : Gain  Gain=Kp_Rvi_pu
  Gain9 : Gain  Gain=DX_DR
  I_thresh : Constant
  Mux2 : Mux  Inputs=2
  Saturation : Saturate  UpperLimit=I_max_VI_pu-1  LowerLimit=0
  Sum1 : Sum  Inputs=-+|
  Sum7 : Sum  Inputs=|+-
  Sum8 : Sum  Inputs=++|
  dq to phasor : Subsystem
  product{,1..3} (4 alike) : Product  InputSameDT=on  RndMeth=Zero  SaturateOnIntegerOverflow=on  OutDataTypeStr=Inherit: Same as first input
  I_rms : Outport  VectorParamsAs1DForOutWhenUnconnected=off
  Delta_E_dq : Outport  Port=2  VectorParamsAs1DForOutWhenUnconnected=off
  wires:
  Sum1/1 -> Saturation/1
  dq to phasor/1(rms) -> Sum1/2, I_rms/1  "I_rms"
  Saturation/1 -> Gain6/1
  I_thresh/1 -> Sum1/1
  Mux2/1 -> Delta_E_dq/1
  Gain6/1 -> product3/2, product/1, product1/2, product2/2
  product3/1 -> Gain5/1
  product/1 -> Gain9/1
  Demux1/1 -> product1/1, product/2  "igd"
  Demux1/2 -> product2/1, product3/1  "igq"
  product1/1 -> Sum7/1
  Gain5/1 -> Sum7/2
  Gain9/1 -> Sum8/1
  product2/1 -> Sum8/2
  Sum7/1 -> Mux2/1
  Sum8/1 -> Mux2/2
  i_VI_dq/1 -> dq to phasor/1(dq_mes), Demux1/1

== system Sim5_MMC/CCSC/Bridge_Model/MMC Average Model/Arm_la ==
  m : Inport
  Controlled Current Source : powerlib/Electrical Sources/Controlled Current Source  Initialize=on  Source_Type=DC  Amplitude=0  Phase=0  Frequency=0  Measurements=None
  Controlled Voltage Source2 : powerlib/Electrical Sources/Controlled Voltage Source  Initialize=on  Source_Type=DC  Amplitude=Vdc/2  Phase=180  Frequency=0  Measurements=None
  Current Measurement7 : spsCurrentMeasurementLib/Current Measurement  PhasorSimulation=off  OutputType=Complex  PSBequivalent=0
  Memory1 : Memory  InitialCondition=Vdc/2
  Memory2 : Memory
  Product : Product  RndMeth=Zero
  Product1 : Product  RndMeth=Zero
  Series RLC Branch : powerlib/Elements/Series RLC Branch  LConnTagsString=__new0  RConnTagsString=__new0  BranchType=C  Resistance=1  Inductance=1e-3  SetiL0=off  InitialCurrent=0  Capacitance=C_arm  Setx0=on  InitialVoltage=Vdc  Measurements=None
  Voltage Measurement : powerlib/Measurements/Voltage Measurement  PhasorSimulation=off  OutputType=Complex  PSBequivalent=0
  Voltage Measurement1 : powerlib/Measurements/Voltage Measurement  PhasorSimulation=off  OutputType=Complex  PSBequivalent=0
  V+ : PMIOPort  Side=Left
  V- : PMIOPort  Port=2  Side=Left
  vctot : Outport
  i_arm : Outport  Port=2
  v_arm : Outport  Port=3
  wires:
  Memory1/1 -> Controlled Voltage Source2/1
  Memory2/1 -> Controlled Current Source/1
  Product/1 -> Memory1/1
  Voltage Measurement/1 -> v_arm/1
  Product1/1 -> Memory2/1
  m/1 -> [m], Product1/1
  Current Measurement7/1 -> i_arm/1, Product1/2
  [m] -> Product/2
  Voltage Measurement1/1 -> Product/1, vctot/1
  connections:
  Current Measurement7/RConn1 -- Controlled Voltage Source2/RConn1
  Current Measurement7/LConn1 -- Voltage Measurement/LConn1 -- V+/RConn1
  Controlled Current Source/LConn1 -- Series RLC Branch/RConn1 -- Voltage Measurement1/LConn2 -- V-/RConn1 -- Voltage Measurement/LConn2 -- Controlled Voltage Source2/LConn1
  Controlled Current Source/RConn1 -- Series RLC Branch/LConn1 -- Voltage Measurement1/LConn1

== system Sim5_MMC/CCSC/Bridge_Model/MMC Average Model/Arm_lb ==
  m : Inport
  Controlled Current Source : powerlib/Electrical Sources/Controlled Current Source  Initialize=on  Source_Type=DC  Amplitude=0  Phase=0  Frequency=0  Measurements=None
  Controlled Voltage Source2 : powerlib/Electrical Sources/Controlled Voltage Source  Initialize=on  Source_Type=DC  Amplitude=Vdc/2  Phase=180  Frequency=0  Measurements=None
  Current Measurement7 : spsCurrentMeasurementLib/Current Measurement  PhasorSimulation=off  OutputType=Complex  PSBequivalent=0
  Memory1 : Memory  InitialCondition=Vdc/2
  Memory2 : Memory
  Product : Product  RndMeth=Zero
  Product1 : Product  RndMeth=Zero
  Series RLC Branch : powerlib/Elements/Series RLC Branch  LConnTagsString=__new0  RConnTagsString=__new0  BranchType=C  Resistance=1  Inductance=1e-3  SetiL0=off  InitialCurrent=0  Capacitance=C_arm  Setx0=on  InitialVoltage=Vdc  Measurements=None
  Voltage Measurement : powerlib/Measurements/Voltage Measurement  PhasorSimulation=off  OutputType=Complex  PSBequivalent=0
  Voltage Measurement1 : powerlib/Measurements/Voltage Measurement  PhasorSimulation=off  OutputType=Complex  PSBequivalent=0
  V+ : PMIOPort  Side=Left
  V- : PMIOPort  Port=2  Side=Left
  vctot : Outport
  i_arm : Outport  Port=2
  v_arm : Outport  Port=3
  wires:
  Memory1/1 -> Controlled Voltage Source2/1
  Memory2/1 -> Controlled Current Source/1
  Product/1 -> Memory1/1
  Voltage Measurement/1 -> v_arm/1
  Product1/1 -> Memory2/1
  m/1 -> [m], Product1/1
  Current Measurement7/1 -> i_arm/1, Product1/2
  [m] -> Product/2
  Voltage Measurement1/1 -> Product/1, vctot/1
  connections:
  Current Measurement7/RConn1 -- Controlled Voltage Source2/RConn1
  Current Measurement7/LConn1 -- Voltage Measurement/LConn1 -- V+/RConn1
  Controlled Current Source/LConn1 -- Series RLC Branch/RConn1 -- Voltage Measurement1/LConn2 -- V-/RConn1 -- Voltage Measurement/LConn2 -- Controlled Voltage Source2/LConn1
  Controlled Current Source/RConn1 -- Series RLC Branch/LConn1 -- Voltage Measurement1/LConn1

== system Sim5_MMC/CCSC/Bridge_Model/MMC Average Model/Arm_lc ==
  m : Inport
  Controlled Current Source : powerlib/Electrical Sources/Controlled Current Source  Initialize=on  Source_Type=DC  Amplitude=0  Phase=0  Frequency=0  Measurements=None
  Controlled Voltage Source2 : powerlib/Electrical Sources/Controlled Voltage Source  Initialize=on  Source_Type=DC  Amplitude=Vdc/2  Phase=180  Frequency=0  Measurements=None
  Current Measurement7 : spsCurrentMeasurementLib/Current Measurement  PhasorSimulation=off  OutputType=Complex  PSBequivalent=0
  Memory1 : Memory  InitialCondition=Vdc/2
  Memory2 : Memory
  Product : Product  RndMeth=Zero
  Product1 : Product  RndMeth=Zero
  Series RLC Branch : powerlib/Elements/Series RLC Branch  LConnTagsString=__new0  RConnTagsString=__new0  BranchType=C  Resistance=1  Inductance=1e-3  SetiL0=off  InitialCurrent=0  Capacitance=C_arm  Setx0=on  InitialVoltage=Vdc  Measurements=None
  Voltage Measurement : powerlib/Measurements/Voltage Measurement  PhasorSimulation=off  OutputType=Complex  PSBequivalent=0
  Voltage Measurement1 : powerlib/Measurements/Voltage Measurement  PhasorSimulation=off  OutputType=Complex  PSBequivalent=0
  V+ : PMIOPort  Side=Left
  V- : PMIOPort  Port=2  Side=Left
  vctot : Outport
  i_arm : Outport  Port=2
  v_arm : Outport  Port=3
  wires:
  Memory1/1 -> Controlled Voltage Source2/1
  Memory2/1 -> Controlled Current Source/1
  Product/1 -> Memory1/1
  Voltage Measurement/1 -> v_arm/1
  Product1/1 -> Memory2/1
  m/1 -> [m], Product1/1
  Current Measurement7/1 -> i_arm/1, Product1/2
  [m] -> Product/2
  Voltage Measurement1/1 -> Product/1, vctot/1
  connections:
  Current Measurement7/RConn1 -- Controlled Voltage Source2/RConn1
  Current Measurement7/LConn1 -- Voltage Measurement/LConn1 -- V+/RConn1
  Controlled Current Source/LConn1 -- Series RLC Branch/RConn1 -- Voltage Measurement1/LConn2 -- V-/RConn1 -- Voltage Measurement/LConn2 -- Controlled Voltage Source2/LConn1
  Controlled Current Source/RConn1 -- Series RLC Branch/LConn1 -- Voltage Measurement1/LConn1

== system Sim5_MMC/CCSC/Bridge_Model/MMC Average Model/Arm_ua ==
  m : Inport
  Controlled Current Source : powerlib/Electrical Sources/Controlled Current Source  Initialize=on  Source_Type=DC  Amplitude=0  Phase=0  Frequency=0  Measurements=None
  Controlled Voltage Source2 : powerlib/Electrical Sources/Controlled Voltage Source  Initialize=on  Source_Type=DC  Amplitude=Vdc/2  Phase=180  Frequency=0  Measurements=None
  Current Measurement7 : spsCurrentMeasurementLib/Current Measurement  PhasorSimulation=off  OutputType=Complex  PSBequivalent=0
  Memory1 : Memory  InitialCondition=Vdc/2
  Memory2 : Memory
  Product : Product  RndMeth=Zero
  Product1 : Product  RndMeth=Zero
  Series RLC Branch : powerlib/Elements/Series RLC Branch  LConnTagsString=__new0  RConnTagsString=__new0  BranchType=C  Resistance=1  Inductance=1e-3  SetiL0=off  InitialCurrent=0  Capacitance=C_arm  Setx0=on  InitialVoltage=Vdc  Measurements=None
  Voltage Measurement : powerlib/Measurements/Voltage Measurement  PhasorSimulation=off  OutputType=Complex  PSBequivalent=0
  Voltage Measurement1 : powerlib/Measurements/Voltage Measurement  PhasorSimulation=off  OutputType=Complex  PSBequivalent=0
  V+ : PMIOPort  Side=Left
  V- : PMIOPort  Port=2  Side=Left
  vctot : Outport
  i_arm : Outport  Port=2
  v_arm : Outport  Port=3
  wires:
  Memory1/1 -> Controlled Voltage Source2/1
  Memory2/1 -> Controlled Current Source/1
  Product/1 -> Memory1/1
  Voltage Measurement/1 -> v_arm/1
  Product1/1 -> Memory2/1
  m/1 -> [m], Product1/1
  Current Measurement7/1 -> i_arm/1, Product1/2
  [m] -> Product/2
  Voltage Measurement1/1 -> Product/1, vctot/1
  connections:
  Current Measurement7/RConn1 -- Controlled Voltage Source2/RConn1
  Current Measurement7/LConn1 -- Voltage Measurement/LConn1 -- V+/RConn1
  Controlled Current Source/LConn1 -- Series RLC Branch/RConn1 -- Voltage Measurement1/LConn2 -- V-/RConn1 -- Voltage Measurement/LConn2 -- Controlled Voltage Source2/LConn1
  Controlled Current Source/RConn1 -- Series RLC Branch/LConn1 -- Voltage Measurement1/LConn1

== system Sim5_MMC/CCSC/Bridge_Model/MMC Average Model/Arm_ub ==
  m : Inport
  Controlled Current Source : powerlib/Electrical Sources/Controlled Current Source  Initialize=on  Source_Type=DC  Amplitude=0  Phase=0  Frequency=0  Measurements=None
  Controlled Voltage Source2 : powerlib/Electrical Sources/Controlled Voltage Source  Initialize=on  Source_Type=DC  Amplitude=Vdc/2  Phase=180  Frequency=0  Measurements=None
  Current Measurement7 : spsCurrentMeasurementLib/Current Measurement  PhasorSimulation=off  OutputType=Complex  PSBequivalent=0
  Memory1 : Memory  InitialCondition=Vdc/2
  Memory2 : Memory
  Product : Product  RndMeth=Zero
  Product1 : Product  RndMeth=Zero
  Series RLC Branch : powerlib/Elements/Series RLC Branch  LConnTagsString=__new0  RConnTagsString=__new0  BranchType=C  Resistance=1  Inductance=1e-3  SetiL0=off  InitialCurrent=0  Capacitance=C_arm  Setx0=on  InitialVoltage=Vdc  Measurements=None
  Voltage Measurement : powerlib/Measurements/Voltage Measurement  PhasorSimulation=off  OutputType=Complex  PSBequivalent=0
  Voltage Measurement1 : powerlib/Measurements/Voltage Measurement  PhasorSimulation=off  OutputType=Complex  PSBequivalent=0
  V+ : PMIOPort  Side=Left
  V- : PMIOPort  Port=2  Side=Left
  vctot : Outport
  i_arm : Outport  Port=2
  v_arm : Outport  Port=3
  wires:
  Memory1/1 -> Controlled Voltage Source2/1
  Memory2/1 -> Controlled Current Source/1
  Product/1 -> Memory1/1
  Voltage Measurement/1 -> v_arm/1
  Product1/1 -> Memory2/1
  m/1 -> [m], Product1/1
  Current Measurement7/1 -> i_arm/1, Product1/2
  [m] -> Product/2
  Voltage Measurement1/1 -> Product/1, vctot/1
  connections:
  Current Measurement7/RConn1 -- Controlled Voltage Source2/RConn1
  Current Measurement7/LConn1 -- Voltage Measurement/LConn1 -- V+/RConn1
  Controlled Current Source/LConn1 -- Series RLC Branch/RConn1 -- Voltage Measurement1/LConn2 -- V-/RConn1 -- Voltage Measurement/LConn2 -- Controlled Voltage Source2/LConn1
  Controlled Current Source/RConn1 -- Series RLC Branch/LConn1 -- Voltage Measurement1/LConn1

== system Sim5_MMC/CCSC/Bridge_Model/MMC Average Model/Arm_uc ==
  m : Inport
  Controlled Current Source : powerlib/Electrical Sources/Controlled Current Source  Initialize=on  Source_Type=DC  Amplitude=0  Phase=0  Frequency=0  Measurements=None
  Controlled Voltage Source2 : powerlib/Electrical Sources/Controlled Voltage Source  Initialize=on  Source_Type=DC  Amplitude=Vdc/2  Phase=180  Frequency=0  Measurements=None
  Current Measurement7 : spsCurrentMeasurementLib/Current Measurement  PhasorSimulation=off  OutputType=Complex  PSBequivalent=0
  Memory1 : Memory  InitialCondition=Vdc/2
  Memory2 : Memory
  Product : Product  RndMeth=Zero
  Product1 : Product  RndMeth=Zero
  Series RLC Branch : powerlib/Elements/Series RLC Branch  LConnTagsString=__new0  RConnTagsString=__new0  BranchType=C  Resistance=1  Inductance=1e-3  SetiL0=off  InitialCurrent=0  Capacitance=C_arm  Setx0=on  InitialVoltage=Vdc  Measurements=None
  Voltage Measurement : powerlib/Measurements/Voltage Measurement  PhasorSimulation=off  OutputType=Complex  PSBequivalent=0
  Voltage Measurement1 : powerlib/Measurements/Voltage Measurement  PhasorSimulation=off  OutputType=Complex  PSBequivalent=0
  V+ : PMIOPort  Side=Left
  V- : PMIOPort  Port=2  Side=Left
  vctot : Outport
  i_arm : Outport  Port=2
  v_arm : Outport  Port=3
  wires:
  Memory1/1 -> Controlled Voltage Source2/1
  Memory2/1 -> Controlled Current Source/1
  Product/1 -> Memory1/1
  Voltage Measurement/1 -> v_arm/1
  Product1/1 -> Memory2/1
  m/1 -> [m], Product1/1
  Current Measurement7/1 -> i_arm/1, Product1/2
  [m] -> Product/2
  Voltage Measurement1/1 -> Product/1, vctot/1
  connections:
  Current Measurement7/RConn1 -- Controlled Voltage Source2/RConn1
  Current Measurement7/LConn1 -- Voltage Measurement/LConn1 -- V+/RConn1
  Controlled Current Source/LConn1 -- Series RLC Branch/RConn1 -- Voltage Measurement1/LConn2 -- V-/RConn1 -- Voltage Measurement/LConn2 -- Controlled Voltage Source2/LConn1
  Controlled Current Source/RConn1 -- Series RLC Branch/LConn1 -- Voltage Measurement1/LConn1

== system Sim5_MMC/CCSC/Control loops/Current Limitation/Current control ==
  Ig_dq0* : Inport
  Ig_dq0 : Inport  Port=2
  vg_dq0 : Inport  Port=3
  w : Inport  Port=4
  Demux : Demux  Outputs=2
  Demux1 : Demux  Outputs=2
  Demux2 : Demux  Outputs=2
  Gain Corrector : Gain  Gain=3/(Tr_I_max/1000)*Lt_pu
  Gain Corrector1 : Gain  Gain=3/(Tr_I_max/1000)*Lt_pu
  Mux : Mux  Inputs=2
  Product : Product  RndMeth=Zero
  Product1 : Product  RndMeth=Zero
  Sum : Sum  Inputs=|+-
  Sum2 : Sum  Inputs=|+-
  Sum3 : Sum  Inputs=|++
  Sum5 : Sum  Inputs=++|
  Sum6 : Sum  Inputs=-+|
  Sum7 : Sum  Inputs=++|
  vpcc_abc{1,3..6} (5 alike) : Scope
  w*Lf_pu : Gain  Gain=Lt_pu
  vm : Outport  InitialOutput=0  VectorParamsAs1DForOutWhenUnconnected=off
  wires:
  Demux2/2 -> Sum7/1
  Demux2/1 -> Sum3/2
  w/1 -> vpcc_abc5/1, w*Lf_pu/1
  Sum/1 -> vpcc_abc1/1, Gain Corrector/1
  Sum7/1 -> Mux/2  "Vm_q*"
  Sum3/1 -> Mux/1, vpcc_abc3/1  "Vm_d*"
  Sum5/1 -> Sum7/2
  Product1/1 -> Sum5/1
  Gain Corrector1/1 -> Sum5/2
  Demux/2 -> Sum6/2
  Sum2/1 -> Sum3/1
  Product/1 -> Sum2/2
  Demux1/2 -> Sum6/1, Product/1
  w*Lf_pu/1 -> Product/2, Product1/1
  Gain Corrector/1 -> Sum2/1
  Demux1/1 -> Sum/2, Product1/2
  Demux/1 -> Sum/1
  Ig_dq0/1 -> Demux1/1
  vg_dq0/1 -> Demux2/1, vpcc_abc6/1
  Sum6/1 -> Gain Corrector1/1
  Ig_dq0*/1 -> vpcc_abc4/1, Demux/1
  Mux/1 -> vm/1

== system Sim5_MMC/CCSC/Control loops/Current Limitation/Inverse Current control ==
  Vm_dq* : Inport
  Ig_dq : Inport  Port=2
  vg_dq : Inport  Port=3
  w : Inport  Port=4
  Demux : Demux  Outputs=2
  Demux1 : Demux  Outputs=2
  Demux2 : Demux  Outputs=2
  Gain Corrector2 : Gain  Gain=1/(3/(Tr_I_max/1000)*Lt_pu)
  Gain Corrector3 : Gain  Gain=1/(3/(Tr_I_max/1000)*Lt_pu)
  Mux : Mux  Inputs=2
  Product : Product  RndMeth=Zero
  Product1 : Product  RndMeth=Zero
  Sum : Sum  Inputs=|+-
  Sum2 : Sum  Inputs=|++
  Sum3 : Sum  Inputs=|++
  Sum5 : Sum  Inputs=-+|
  Sum6 : Sum  Inputs=-+|
  Sum7 : Sum  Inputs=++|
  w*Lf_pu : Gain  Gain=Lt_pu
  Is_dq* : Outport  InitialOutput=0  VectorParamsAs1DForOutWhenUnconnected=off
  wires:
  vg_dq/1 -> Demux2/1
  Ig_dq/1 -> Demux1/1
  Vm_dq*/1 -> Demux/1
  Demux/1 -> Sum/1
  Demux1/1 -> Sum3/2, Product1/2
  Sum/1 -> Sum2/1
  w*Lf_pu/1 -> Product1/1, Product/2
  Product/1 -> Sum2/2
  Sum2/1 -> Gain Corrector3/1
  Mux/1 -> Is_dq*/1
  Demux/2 -> Sum6/2
  Sum6/1 -> Sum5/2
  Sum5/1 -> Gain Corrector2/1
  Sum3/1 -> Mux/1  "is_d*"
  Sum7/1 -> Mux/2  "is_q*"
  w/1 -> w*Lf_pu/1
  Demux1/2 -> Sum7/1, Product/1
  Gain Corrector3/1 -> Sum3/1
  Demux2/1 -> Sum/2
  Demux2/2 -> Sum6/1
  Product1/1 -> Sum5/1
  Gain Corrector2/1 -> Sum7/2
